simulink model "SIM_EXO_DAL"  (R2021b)
(part 18 of 25)

et753 = t4.*t5.*t7.*1.873025744810486e-7-t4.*t7.*t9.*3.446085442739697e-7;
et754 = t91.*t5684.*t6216.*1.656182742171539e-72;
et755 = t91.*t5824.*t6213.*(-1.656182742171539e-72);
et756 = t5684.*t6230.*(t29-t30).*(-1.656182742171539e-72);
et757 = t5824.*t6222.*(t29-t30).*1.656182742171539e-72;
et758 = t4.*8.79383415291399e-9-t8.*1.262353016789131e-9+(t6401.*(t5808-t6019+t5679.*(t2088-t4743).*3.038581678643136e-64))./2.0;
et759 = t5.*t8.*2.179051830709965e-7-t8.*t72-(t4.*t640)./2.0-t8.*t1496+(t5.*t3443)./2.0-(t9.*t3514)./2.0-(t615.*t6422)./2.0;
et760 = (t6359.*(t5831-t6095+t5679.*(t2088-t4743).*8.081970098144003e-70))./2.0+(t8.*t9.*t1460)./2.0;
et761 = t4.*(-3.403234468928681e-8);
et762 = t202.*1.910352536348279e-6;
et763 = t7.*t8.*5.724235841753608e-8;
et764 = t4.*t190.*1.109465165290797e-6-t9.*t5657.*4.00912737776847e-7+t112.*t5657;
et765 = t5.*t6349.*(-7.01299275e-12)-t9.*t6350.*7.01299275e-12+(t5.*t7042)./2.0+(t9.*t7045)./2.0+t1489.*t5657-(t1426.*t5939)./2.0-(t5658.*t6405)./2.0+(t5662.*t6402)./2.0-(t5939.*t6399)./2.0+(t5940.*t6400)./2.0+(t6422.*t7012)./2.0-(t640.*(t2421-t4158))./2.0-(t5.*t1471.*t5657)./2.0;
et766 = t3.*t8.*t34.*t191.*2.142628988669224e-22;
et767 = t263-t300-t373+t377+t395-t402+t431-t441+t442-t454-t457-t481+t482-t489+t491-t494+t496+t516+t517-t540+t559+t563+t564-t568-t582+t584+t605+t614-t625-t911-t971-t986+t1282-t1670+t4089+t4123+t7221+t7223;
et768 = (t1426.*(-t5881+t5918+t6412+t6414+(t4.*t5824.*t5861.*(t29-t30))./1.316403645856965e+67+(t4.*t91.*t5824.*(t3136-t5691))./1.316403645856965e+67))./2.0;
et769 = t3.*t8.*5.337065020227051e-7-t3.*t5.*t8.*1.873025744810486e-7;
et770 = t5.*t7.*t9.*t18.*(-1.07175327657342e-6);
et771 = t199.*4.620317820983189e-6+t753+t797+t848+t852+t902+t908+t917+t928+t931+t944+t952+t975+t976+t991+t1090+t1122+t1147+t1156+t1194+t1292+t1441+t1816+t2028+t2486+t3416+t3417+t3426+t3429+t3432+t3464+t3465+t3469+t3489+t3498+t3501+t3504+t3510+t3521+t3530+t3535+t3540+t3554+t3571+t3574+t3577+t3578+t3605+t3607+t3637+t3659+t3666+t3694+t3726+t3863+t3960+t4004+t4011+t4015;
et772 = t4134+t4423+t4592+t4780-t5621-t5847-t5849-t5982+t6360-t6362-t6442+t6445-t6451-t6563-t6564+t6879+t7006+t7008+t7022+t7023+t3.*t4.*1.384445455377623e-7;
et773 = t4.*t7.*t34.*t191.*(-5.182094253151392e-22);
et774 = (t6401.*(t5808-t6019+t5679.*(t2088-t4743).*3.038581678643136e-64))./2.0;
et775 = (t6359.*(t5831-t6095+t5679.*(t2088-t4743).*8.081970098144003e-70))./2.0;
et776 = t5888+t5795.*(t2088-t4743).*8.081970098144003e-70;
et777 = t5683.*(t197.*(t29-t30).*9.007199254740992e+15+t3.*(t2444-t2449)).*8.081970098144003e-70;
et778 = t5842+t5795.*(t2088-t4743).*3.038581678643136e-64;
et779 = t5683.*(t197.*(t29-t30).*9.007199254740992e+15+t3.*(t2444-t2449)).*3.038581678643136e-64;
et780 = t201.*8.987911871652987e-9+t202.*6.359001115808088e-7-t1542+t1551+t1627+t1648+t1710+t1732+t1806-t1855+t1922+t1947-t1986+t2002+t2017+t2035-t2062-t2123+t2143-t2181-t2187+t2192-t2196-t2202;
et781 = -t2213-t2289+t2303-t2312+t2314+t2338-t2392+t2397+t2465+t2524-t2530+t2539+t2554+t2556+t2560+t2627+t4279+t4395+t4406+t4416+t4426+t4462-t4469+t4490-t4520+t4545-t4551+t4558-t4559+t4575-t4581+t4588+t4589-t4590-t4591-t4605-t4607-t4614+t4616-t4622+t4626+t4666-t4667-t4669+t4675-t4694+t4695-t4697+t4708-t4724-t4732-t4745+t4747-t4755+t4756+t4782+t4785-t4786;
et782 = t4.*t190.*1.069583140309415e-6-t5.*t201.*1.608000198040319e-13;
et783 = t5.*t202.*(-2.227142959217101e-7)+t9.*t201.*2.10868590222219e-13;
et784 = t19.*t202.*(-1.274380648825446e-6)+t202.*t240+t23.*t1551+t23.*t1627+t5.*t1687-t4.*t5.*t190.*3.746051489620971e-7;
et785 = t4.*t9.*t190.*6.892170885479394e-7-t8.*t9.*t190.*3.546806877605634e-13;
et786 = t4.*t19.*t190.*(-2.143506553146841e-6)+t5.*t9.*t202.*8.376559107229145e-7;
et787 = t4.*t34.*t191.*(-3.795202701448175e-22);
et788 = t8.*t34.*t191.*2.95048074153502e-22;
et789 = t19.*t23.*t196.*(-4.188279553614573e-7)+t4.*t5.*t9.*t190.*1.408936125616489e-6;
et790 = t5.*t8.*t17.*t190.*(-2.7046541903611e-13);
et791 = t3.*t4.*t34.*t191.*5.099405807101157e-25;
et792 = t5.*t9.*t23.*t196.*(-6.371903244127231e-7);
et793 = t3.*t8.*t34.*t191.*3.607859943485489e-23;
et794 = t4.*t7.*t34.*t191.*4.962704675595027e-22;
et795 = t5.*t8.*t34.*t191.*3.738830062544659e-22;
et796 = t7.*t8.*t34.*t191.*6.383525886533628e-22;
et797 = t8.*t9.*t34.*t191.*2.032139097819379e-22;
et798 = t3.*t4.*t5.*t34.*t191.*(-9.123193089563036e-30);
et799 = t3.*t4.*t9.*t34.*t191.*1.196389694146674e-29;
et800 = t3.*t5.*t8.*t34.*t191.*(-1.263597807995354e-23);
et801 = t4.*t5.*t7.*t34.*t191.*6.288707183017346e-22;
et802 = t3.*t8.*t9.*t34.*t191.*2.324829770052718e-23;
et803 = t4.*t7.*t9.*t34.*t191.*3.418055254602648e-22;
et804 = t3.*t8.*t19.*t34.*t191.*(-7.230360259287513e-23);
et805 = t3.*t4.*t5.*t7.*t34.*t191.*(-2.125369829239315e-23);
et806 = t3.*t5.*t8.*t9.*t34.*t191.*4.752547061531711e-23;
et807 = t5961-t6215-t6473+(t91.*t5824.*(t5670+t4.*(t1458-t5665)))./1.316403645856965e+67+(t5824.*t6103.*(t29-t30))./1.316403645856965e+67;
et808 = (t5822.*t6230.*(t29-t30))./1.316403645856965e+67;
et809 = t5889+t5795.*(t2088-t4743).*5.344156668414146e-72;
et810 = t5683.*(t197.*(t29-t30).*9.007199254740992e+15+t3.*(t2444-t2449)).*5.344156668414146e-72;
et811 = t5888+t5795.*(t2088-t4743).*8.081970098144003e-70;
et812 = t5683.*(t197.*(t29-t30).*9.007199254740992e+15+t3.*(t2444-t2449)).*8.081970098144003e-70;
et813 = t5892+t5795.*(t2088-t4743).*7.671525497590686e-73;
et814 = t5683.*(t197.*(t29-t30).*9.007199254740992e+15+t3.*(t2444-t2449)).*7.671525497590686e-73;
et815 = t6008+t6123-t6672+(t5684.*t6468.*(t29-t30))./1.316403645856965e+67-(t5.*t91.*t5824.*t6216)./1.316403645856965e+67;
et816 = (t5.*t5824.*t6230.*(t29-t30))./1.316403645856965e+67;
et817 = t5882+t5795.*(t2088-t4743).*1.879526485671887e-68;
et818 = t5683.*(t197.*(t29-t30).*9.007199254740992e+15+t3.*(t2444-t2449)).*1.879526485671887e-68;
et819 = t5883+t5795.*(t2088-t4743).*4.121912899099809e-68;
et820 = t5683.*(t197.*(t29-t30).*9.007199254740992e+15+t3.*(t2444-t2449)).*4.121912899099809e-68;
et821 = t741+t868+t1568+t1834-t3274-t3391-t3440+t3874+t3891+t4348+t5259+t5742+t5757-t5.*t8.*1.133811468776912e-7;
et822 = t5.*t201.*(-6.364473664374288e-6)+t8.*t3365+t8.*t3449;
et823 = t4.*t5.*t7.*(-1.907069379620846e-7);
et824 = t8.*t9.*t190.*(-6.800564119502148e-6);
et825 = t3.*t4.*t5.*t34.*t191.*(-7.138318981153782e-22);
et826 = t199.*(-2.737706926505492e-6)+t1541+t1570+t1607-t1609-t1616+t1656+t1747-t1783+t1792-t1805+t1908-t2795+t4181+t4221-t4228+t4342-t4344+t4345-t4403+t4413-t4431-t4495+t4501-t4502+t4509+t4919+t4983-t5769+t5921+t5922+t6119+t6406-t6407+t6443-t6477+t6489+t6593-t6594-t7051-t7054;
et827 = -t7088+t7091+t7114-t7115+t7174+t7261-t7322+(t5658.*(et809+et810))./2.0+(t6776.*(t6313+(t91.*t5824.*(t6218+t5.*(t3136-t5691)))./1.316403645856965e+67+(t5824.*t6470.*(t29-t30))./1.316403645856965e+67))./2.0;
et828 = (t4119.*(et811+et812))./2.0+(t5662.*(et813+et814))./2.0+(t7027.*(et815+et816))./2.0+(t5940.*(et817+et818))./2.0+(t5939.*(et819+et820))./2.0+(t318.*(et821+et822+et823+et824+et825))./2.0-t4.*t17.*t190.*2.170136264005124e-9;
et829 = t8.*t34.*t191.*(-3.477878712271355e-22);
et830 = t4.*t7.*t34.*t191.*9.787964718254394e-24;
et831 = dq5.*((t6359.*(et776+et777))./2.0+(t6401.*(et778+et779))./2.0)-dq1.*(et780+et781+et782+et783+et784+et785+et786+et787+et788+et789+et790+et791+et792+et793+et794+et795+et796+et797+et798+et799+et800+et801+et802+et803+et804+et805+et806)+dq6.*(t3142-t4099-t4103+t4810-t4904+t7066+t7074+t7307+t7308+t7376+t7377+t7380+t7427+t7428+t7447+t7448+t7468+t7477+t7491+t7492+t7493);
et832 = -dq3.*(t922+t934+t940+t989+t1039+t1050+t1056+t1069+t1083+t1099+t1106+t1133+t1150+t1177+t1179+t1185+t1191+t1196+t1205+t1221+t1225+t1233+t1250+t1253+t1273+t1274+t1306+t1316+t1322+t1330+t1331+t1337+t1342+t1348+t1353+t1379+t1391+t1402+t1407+t1411+t1413+t1419+t1423+t1436+t1443+t1445+t1454+t1457+t1486+t1487+t1767+t1827+t1873+t1992+t2130+t2180+t2474+t2481+t5.*t7274.*1.40259855e-11-t9.*t7276.*1.40259855e-11+t1426.*(et807+et808))+dq2.*(et826+et827+et828+et829+et830);
et833 = -dq4.*(t290+t357+t406+t411+t418+t423+t424+t429+t440+t449+t479+t480+t483+t488+t492+t532+t540+t545+t580+t581+t590+t604+t611+t618+t623+t911+t971+t986+t1324+t1670+t4100+t4132+t7143+t7222+t7224);
et834 = -t235+t315+t413+t539+t543+t567+t6081-t6167+t6182+t6521+t6537-t6677+t5704.*t5784+t91.*t5684.*(t6218+t5.*(t3136-t5691)).*1.015171749786156e-71;
et835 = t5684.*t6468.*(t29-t30).*5.517689141340903e-72;
et836 = t5684.*t6470.*(t29-t30).*1.015171749786156e-71;
et837 = t5.*t91.*t5824.*t6216.*(-5.517689141340903e-72);
et838 = t5.*t5824.*t6230.*(t29-t30).*5.517689141340903e-72;
et839 = t284-t311+t391-t463+t534+t5947-t6009.*1.40259855e-11+t6013.*7.26350610236655e-5-t6194+t6449+t6454-t6513+t6544+t6551;
et840 = t91.*t5684.*(t6218+t5.*(t3136-t5691)).*1.065477564130357e-78-t4.*t7.*t9.*1.07175327657342e-6;
et841 = t5824.*t6222.*(t29-t30).*5.517689141340903e-72;
et842 = t5684.*t6470.*(t29-t30).*1.065477564130357e-78;
et843 = t741+t868+t1568+t1834-t3274-t3391-t3440+t3874+t3891+t4348+t5259+t5742+t5757-t5.*t8.*1.133811468776912e-7;
et844 = t5.*t201.*(-6.364473664374288e-6)+t8.*t3365+t8.*t3449;
et845 = t4.*t5.*t7.*(-1.907069379620846e-7);
et846 = t8.*t9.*t190.*(-6.800564119502148e-6);
et847 = t3.*t4.*t5.*t34.*t191.*(-7.138318981153782e-22);
et848 = dq3.*(t3142+t4108+t4115+t4810+t4984+t7066+t7074+t7307+t7308+t7414+t7442+t7444+t7504+(t6821.*(et834+et835+et836+et837+et838))./2.0+(t7130.*(et839+et840+et841+et842))./2.0)-dq4.*(t622+t632+t712+t1503+t1523+t6941+t7059+t7081+t7136+t7137+t7201+t7203+t7272+t7273)+dq5.*(-t72+t112+t616+t619-t1489+t1496)+dq6.*(-t7459-t7501+t7502+t7508-t7541-t7542+t638.*t6821+t594.*t7129+t600.*t7130-t1460.*t7130+t1471.*t7129)+dq2.*(t5797+t5926+t5928+t5937+t5938+t6271+t7231+t7235-t7271-t7343+t7344+(t6821.*(et843+et844+et845+et846+et847))./2.0);
et849 = -dq1.*(t684+t781+t792+t803+t826+t832+t875+t893+t912+t915+t1088+t1201+t1612+t1734+t1740+t1814+t1833+t1968+t1997+t2004+t2069+t2115+t2133+t2267+t3338+t3375+t3390+t3392+t3400+t3420+t3422+t3435+t3437+t3439+t3446+t3458+t3474+t3483+t3491+t3547+t3556+t3610+t3662+t3706+t3755+t3763+t3792+t3822+t3831+t3852+t3873+t3951+t3957+t3979+t3993+t4249+t4304+t4347+t4447+t4527+t4587+t7257-t7341-t7342+t7405-t7431-t7434);
et850 = t5889+t5795.*(t2088-t4743).*5.344156668414146e-72;
et851 = t5683.*(t197.*(t29-t30).*9.007199254740992e+15+t3.*(t2444-t2449)).*5.344156668414146e-72;
et852 = t5888+t5795.*(t2088-t4743).*8.081970098144003e-70;
et853 = t5683.*(t197.*(t29-t30).*9.007199254740992e+15+t3.*(t2444-t2449)).*8.081970098144003e-70;
et854 = t5892+t5795.*(t2088-t4743).*7.671525497590686e-73;
et855 = t5683.*(t197.*(t29-t30).*9.007199254740992e+15+t3.*(t2444-t2449)).*7.671525497590686e-73;
et856 = -t231+t275+t469+t553+t6074+t6175-t6676+t5.*t6536+t5684.*t6468.*(t29-t30).*5.520609140571798e-70;
et857 = t5.*t91.*t5824.*t6216.*(-5.520609140571798e-70);
et858 = t5882+t5795.*(t2088-t4743).*1.879526485671887e-68;
et859 = t5683.*(t197.*(t29-t30).*9.007199254740992e+15+t3.*(t2444-t2449)).*1.879526485671887e-68;
et860 = t5883+t5795.*(t2088-t4743).*4.121912899099809e-68;
et861 = t5683.*(t197.*(t29-t30).*9.007199254740992e+15+t3.*(t2444-t2449)).*4.121912899099809e-68;
et862 = -dq1.*(t7558-t7574+dq6.*t7104+dq4.*t7256-dq3.*t7595)+dq5.*(-dq6.*(et735+et736+et737)+dq3.*(et748+et749+et750+et751+et752+et753+et754+et755+et756+et757)+dq4.*(et758+et759+et760)+dq2.*(et761+et762+et763+et764+et765+et766));
et863 = -dq4.*(t5825+t7258+dq2.*(et771+et772+et773)+dq6.*(t622-t624-t681+t1503+t1523+t7059+t7206+t7272+t7273+t7348-t7350+t7367-t7369+t7371-t7485+t7487-t7490+t4.*t9.*(t5709-t6255+t6282+t6296-t7003+t6216.*(t6218+t5.*(t3136-t5691)).*1.40259855e-11).*(3.0./1.0e+3))-dq3.*(et767+et768+et769+et770)-dq5.*(et774+et775))+dq3.*(et831+et832+et833)+dq6.*(et848+et849);
et864 = dq2.*(-t7557-t7558+dq4.*t7572+dq6.*t7597+dq3.*(-t5769+t5921+t5922+t5958-t5960+t5974+t5978+t6119+t6202+t6203+t6209+t6210-t6329+t6330+t6406-t6407+t6443-t6477+t6489+t6593-t6594-t7102+t7156-t7158+t7217+t7277+t7279+t7300+t7321+t7435+t7437+t7455+(t5658.*(et850+et851))./2.0+(t4119.*(et852+et853))./2.0+(t5662.*(et854+et855))./2.0+(t6462.*(et856+et857))./2.0+(t5940.*(et858+et859))./2.0+(t5939.*(et860+et861))./2.0));
et865 = t6191.*(-2.179051830709965e-7)+t6197.*4.00912737776847e-7+t6930.*4.00912737776847e-7+t6937.*4.00912737776847e-7;
et866 = t6939.*(-2.179051830709965e-7)-t7459-t7501+t7502+t7508-t7541-t7542+t6216.*(t6218+t5.*(t3136-t5691)).*2.179051830709965e-7+(t9.*(-t6235+t6248+t6952+t6983-t6989+t6216.*(t6218+t5.*(t3136-t5691)).*1.744166498897461e-6))./2.0-(t5.*t7366)./2.0+(t638.*t6821)./2.0;
et867 = (t594.*t7129)./2.0+(t600.*t7130)./2.0-(t1460.*t7130)./2.0+(t1471.*t7129)./2.0+(t9.*(-t5744+t6232+t6248+t6303+t6322+t6952+t6960+t6983+t6991))./2.0+(t5.*(t6197.*3.383302988283333e-6-t6231+t6954+t6985-t6990+t6216.*(t6218+t5.*(t3136-t5691)).*1.246862701090643e-6))./2.0;
et868 = ((t4148+t5.*(t2421-t4158)).*(-t6235+t6248+t6952+t6983-t6989+t6216.*(t6218+t5.*(t3136-t5691)).*1.744166498897461e-6))./2.0-(t5657.*t7331)./2.0-(t5872.*t7366)./2.0-(t6462.*t7133)./2.0+(t6463.*t7134)./2.0+(t6462.*t7204)./2.0-(t6821.*t7098)./2.0+(t7032.*t7129)./2.0-(t7033.*t7130)./2.0-(t7082.*t7130)./2.0+(t7085.*t7129)./2.0+((t4148+t5.*(t2421-t4158)).*(-t5744+t6232+t6248+t6303+t6322+t6952+t6960+t6983+t6991))./2.0;
et869 = (t6136.*(t6197.*1.33637579258949e-4-t6225+t6944+t6975-t6986+t6216.*(t6218+t5.*(t3136-t5691)).*7.26350610236655e-5))./2.0+(t6463.*(t5709-t6255+t6282+t6296-t7003+t6216.*(t6218+t5.*(t3136-t5691)).*1.40259855e-11))./2.0;
et870 = (t5872.*(t6197.*3.383302988283333e-6-t6231+t6954+t6985-t6990+t6216.*(t6218+t5.*(t3136-t5691)).*1.246862701090643e-6))./2.0;
et871 = (t7130.*(-t6235+t6248+t6952+t6983-t6989+t6216.*(t6218+t5.*(t3136-t5691)).*1.744166498897461e-6))./2.0-(t6821.*t7331)./2.0-(t7129.*t7366)./2.0+(t7130.*(-t5744+t6232+t6248+t6303+t6322+t6952+t6960+t6983+t6991))./2.0;
et872 = (t7129.*(t6197.*3.383302988283333e-6-t6231+t6954+t6985-t6990+t6216.*(t6218+t5.*(t3136-t5691)).*1.246862701090643e-6))./2.0;
et873 = t6313+(t91.*t5824.*(t6218+t5.*(t3136-t5691)))./1.316403645856965e+67+(t5824.*t6470.*(t29-t30))./1.316403645856965e+67;
et874 = (t5709-t6255+t6282+t6296-t7003+t6216.*(t6218+t5.*(t3136-t5691)).*1.40259855e-11)./2.0;
et875 = t7453+t7529+t7530+t7552+t7562+t7563+(t7133.*(-t6729+t5784.*(t4148+t5.*(t2421-t4158))+(t5824.*t6468.*(t29-t30))./1.316403645856965e+67))./2.0;
et876 = t7204.*(-t6729+t5784.*(t4148+t5.*(t2421-t4158))+(t5824.*t6468.*(t29-t30))./1.316403645856965e+67).*(-1.0./2.0);
et877 = (t7134.*(t6313+(t91.*t5824.*(t6218+t5.*(t3136-t5691)))./1.316403645856965e+67+(t5824.*t6470.*(t29-t30))./1.316403645856965e+67))./2.0;
et878 = (t1427.*(-t6235+t6248+t6952+t6983-t6989+t6216.*(t6218+t5.*(t3136-t5691)).*1.744166498897461e-6))./2.0+(t318.*t7331)./2.0-(t1429.*t7366)./2.0+(t6821.*t7309)./2.0-(t7124.*t7130)./2.0-(t7130.*t7267)./2.0-(t7129.*t7269)./2.0;
et879 = (t7129.*(t305-t319+t322+t336+t6345+t6807+t6818-t5.*t7.*t8.*2.908151843953269e-6-t7.*t8.*t9.*1.07175327657342e-6))./2.0+(t1427.*(-t5744+t6232+t6248+t6303+t6322+t6952+t6960+t6983+t6991))./2.0+et873.*et874;
et880 = ((t6005-t6486+(t5824.*t6230.*(t29-t30))./1.316403645856965e+67).*(t6197.*1.33637579258949e-4-t6225+t6944+t6975-t6986+t6216.*(t6218+t5.*(t3136-t5691)).*7.26350610236655e-5))./2.0;
et881 = (t1429.*(t6197.*3.383302988283333e-6-t6231+t6954+t6985-t6990+t6216.*(t6218+t5.*(t3136-t5691)).*1.246862701090643e-6))./2.0;
et882 = t738+t910+t930+t1019+t1077+t1212+t1659+t1835+t1938+t2052+t3457+t3479+t3542+t3584+t3612+t3667+t3732+t3875+t3922+t3968+t4286+t4349+t4370+t4553-t4.*t5.*1.043021220661002e-7;
et883 = t4.*t9.*(-5.669057343884558e-8)+t8.*t1798+t8.*t2083+t8.*t4183+t8.*t4208+t8.*t4259+t8.*t4337-(t6821.*t7297)./2.0+(t7129.*t7141)./2.0-(t7130.*t7140)./2.0+(t7130.*t7244)./2.0+(t7129.*t7248)./2.0;
et884 = t2.*t3.*t5.*(-3.337218585173762e-6);
et885 = t2.*t4.*t5.*(-3.65040710056658e-6);
et886 = t2.*t3.*t9.*6.139979878798348e-6;
et887 = t3.*t5.*t6.*8.090164539562037e-7;
et888 = t2.*t4.*t9.*(-1.984079208716435e-6);
et889 = t4.*t5.*t6.*8.849403575532204e-7;
et890 = t3.*t6.*t9.*(-1.488468502176114e-6);
et891 = t4.*t6.*t9.*4.809851931591181e-7;
et892 = t4.*t5.*t190.*3.400282059751074e-6;
et893 = t2.*t5.*t196.*(-4.809851931591181e-7);
et894 = t4.*t9.*t190.*1.848130565348858e-6;
et895 = t2.*t9.*t196.*8.849403575532204e-7;
et896 = t5.*t6.*t196.*(-1.984079208716435e-6);
et897 = t2.*t5.*t202.*8.849403575532204e-7;
et898 = t6.*t9.*t196.*3.65040710056658e-6;
et899 = t2.*t9.*t202.*4.809851931591181e-7;
et900 = t5.*t6.*t202.*3.65040710056658e-6;
et901 = t6.*t9.*t202.*1.984079208716435e-6;
et902 = t5.*t6.*t7.*t8.*(-1.488468502176114e-6);
C_dq = ft_17({dq1,dq2,dq3,dq4,dq5,dq6,et294,et295,et296,et341,et342,et343,et627,et628,et629,et630,et732,et733,et734,et862,et863,et864,et865,et866,et867,et868,et869,et870,et871,et872,et875,et876,et877,et878,et879,et880,et881,et882,et883,et884,et885,et886,et887,et888,et889,et890,et891,et892,et893,et894,et895,et896,et897,et898,et899,et900,et901,et902,t1004,t1016,t1031,t1061,t1075,t1081,t1095,t1101,t1108,t113,t1144,t115,t1152,t1155,t1170,t1171,t1174,t1184,t1193,t1203,t1207,t1213,t1215,t1224,t1227,t1245,t125,t1254,t1258,t1285,t1288,t1300,t1301,t131,t132,t1323,t1333,t1344,t1345,t1365,t1377,t1380,t1383,t1388,t1409,t1427,t1428,t1429,t144,t1440,t1458,t148,t1489,t150,t1503,t1508,t1523,t1537,t1540,t156,t158,t1593,t1621,t1622,t1642,t1661,t1672,t1692,t17,t1704,t171,t1715,t1719,t1721,t1731,t1759,t1769,t1770,t1775,t1777,t18,t1831,t1847,t185,t1858,t1870,t19,t190,t191,t196,t1977,t1981,t1984,t199,t2,t2014,t2034,t2043,t2096,t2121,t2132,t2150,t2165,t2177,t2184,t2203,t2236,t2333,t2341,t2383,t2390,t2395,t24,t2421,t2546,t257,t258,t277,t278,t287,t29,t3,t30,t302,t309,t3136,t3142,t318,t3321,t34,t3407,t3409,t3430,t3444,t3450,t3463,t3468,t3475,t3485,t3490,t3496,t3499,t3507,t3513,t3515,t3522,t3523,t3526,t3531,t3543,t356,t3569,t358,t3583,t3585,t3606,t361,t3618,t3658,t371,t3719,t372,t3734,t3738,t374,t3757,t3788,t379,t3843,t3869,t3871,t3992,t4,t4099,t4103,t4148,t4153,t4158,t4179,t4185,t4190,t422,t4230,t4232,t4254,t4255,t427,t428,t4317,t433,t434,t436,t4369,t4396,t4397,t4412,t4417,t4419,t4420,t4428,t4429,t4436,t444,t4440,t445,t4478,t448,t4485,t4506,t4519,t452,t4522,t453,t4530,t4541,t4549,t4556,t4557,t4568,t4572,t458,t4596,t460,t4619,t4625,t4648,t4656,t4660,t4727,t4733,t4739,t475,t477,t4810,t485,t486,t4904,t493,t5,t508,t510,t512,t514,t520,t522,t524,t5275,t533,t535,t547,t561,t5665,t5666,t5670,t5676,t5691,t5709,t5718,t5730,t5738,t5744,t5784,t5822,t5824,t5845,t586,t5861,t587,t5878,t5905,t592,t5942,t5943,t5944,t5951,t5954,t596,t5961,t5967,t5973,t6,t6005,t6026,t603,t6035,t6037,t6042,t6044,t6046,t6047,t6048,t6053,t6056,t6060,t610,t6103,t6118,t612,t6142,t6145,t6146,t6147,t6152,t6155,t6158,t6162,t6164,t6165,t6170,t6171,t6177,t6179,t6183,t6189,t6195,t6196,t6197,t620,t621,t6213,t6215,t6216,t6218,t622,t6220,t6226,t6230,t6231,t6232,t6235,t6239,t6244,t6248,t6249,t6252,t6255,t6276,t6282,t6289,t6293,t6296,t6303,t6307,t6312,t6313,t632,t6322,t6352,t6465,t6468,t6470,t6473,t6486,t6487,t6546,t6548,t6557,t6562,t6604,t6605,t6607,t6648,t6656,t6711,t6714,t6715,t6721,t6724,t6727,t6729,t6738,t6743,t6746,t6747,t6753,t6756,t6758,t6821,t6831,t6838,t6841,t6842,t6844,t6847,t6849,t6851,t6856,t6859,t6860,t6865,t6884,t6888,t6890,t6891,t6892,t6894,t6898,t6903,t6909,t6911,t6914,t6915,t6916,t6918,t6921,t6922,t6924,t6928,t6935,t6936,t6946,t6952,t6953,t6954,t6960,t6977,t6983,t6984,t6985,t6989,t6990,t6991,t6994,t7,t7000,t7003,t7026,t7035,t7036,t7039,t7040,t7084,t7086,t7087,t7095,t7096,t7100,t7103,t7104,t712,t7127,t7128,t7129,t7130,t7133,t7134,t7194,t72,t7204,t7206,t7207,t7208,t724,t7242,t7243,t7245,t7246,t7247,t7254,t7255,t7268,t7270,t7274,t7276,t73,t7327,t7331,t7332,t7336,t7340,t7346,t7348,t7349,t7350,t7362,t7363,t7366,t7367,t7368,t7369,t7371,t7372,t7373,t7374,t7375,t7376,t7377,t7378,t7379,t7380,t7381,t7382,t7383,t7384,t7385,t7390,t7391,t7392,t7393,t7394,t7395,t7396,t7398,t7399,t7402,t7403,t742,t7423,t7425,t7426,t7427,t7428,t7429,t7430,t7433,t7439,t7440,t7446,t7447,t7448,t7453,t7459,t7463,t7468,t7476,t7477,t7481,t7482,t7485,t7486,t7487,t7488,t7490,t7491,t7492,t7493,t7496,t7498,t7499,t7500,t7501,t7503,t7507,t7509,t7510,t7511,t7512,t7513,t7515,t7516,t7517,t7519,t7521,t7522,t7523,t7524,t7525,t7526,t7527,t7529,t7530,t7531,t7533,t7534,t7536,t7537,t7538,t7541,t7542,t7543,t7546,t7548,t7549,t7550,t7552,t7554,t7555,t7562,t7563,t7565,t7587,t7597,t7599,t8,t825,t827,t845,t866,t869,t874,t877,t881,t899,t9,t90,t903,t91,t919,t926,t932,t947,t957,t958,t968,t970,t972,t984,t985,t998});
end
function C_dq = ft_17(ct)
dq1 = ct{1};
dq2 = ct{2};
dq3 = ct{3};
dq4 = ct{4};
dq5 = ct{5};
dq6 = ct{6};
et294 = ct{7};
et295 = ct{8};
et296 = ct{9};
et341 = ct{10};
et342 = ct{11};
et343 = ct{12};
et627 = ct{13};
et628 = ct{14};
et629 = ct{15};
et630 = ct{16};
et732 = ct{17};
et733 = ct{18};
et734 = ct{19};
et862 = ct{20};
et863 = ct{21};
et864 = ct{22};
et865 = ct{23};
et866 = ct{24};
et867 = ct{25};
et868 = ct{26};
et869 = ct{27};
et870 = ct{28};
et871 = ct{29};
et872 = ct{30};
et875 = ct{31};
et876 = ct{32};
et877 = ct{33};
et878 = ct{34};
et879 = ct{35};
et880 = ct{36};
et881 = ct{37};
et882 = ct{38};
et883 = ct{39};
et884 = ct{40};
et885 = ct{41};
et886 = ct{42};
et887 = ct{43};
et888 = ct{44};
et889 = ct{45};
et890 = ct{46};
et891 = ct{47};
et892 = ct{48};
et893 = ct{49};
et894 = ct{50};
et895 = ct{51};
et896 = ct{52};
et897 = ct{53};
et898 = ct{54};
et899 = ct{55};
et900 = ct{56};
et901 = ct{57};
et902 = ct{58};
t1004 = ct{59};
t1016 = ct{60};
t1031 = ct{61};
t1061 = ct{62};
t1075 = ct{63};
t1081 = ct{64};
t1095 = ct{65};
t1101 = ct{66};
t1108 = ct{67};
t113 = ct{68};
t1144 = ct{69};
t115 = ct{70};
t1152 = ct{71};
t1155 = ct{72};
t1170 = ct{73};
t1171 = ct{74};
t1174 = ct{75};
t1184 = ct{76};
t1193 = ct{77};
t1203 = ct{78};
t1207 = ct{79};
t1213 = ct{80};
t1215 = ct{81};
t1224 = ct{82};
t1227 = ct{83};
t1245 = ct{84};
t125 = ct{85};
t1254 = ct{86};
t1258 = ct{87};
t1285 = ct{88};
t1288 = ct{89};
t1300 = ct{90};
t1301 = ct{91};
t131 = ct{92};
t132 = ct{93};
t1323 = ct{94};
t1333 = ct{95};
t1344 = ct{96};
t1345 = ct{97};
t1365 = ct{98};
t1377 = ct{99};
t1380 = ct{100};
t1383 = ct{101};
t1388 = ct{102};
t1409 = ct{103};
t1427 = ct{104};
t1428 = ct{105};
t1429 = ct{106};
t144 = ct{107};
t1440 = ct{108};
t1458 = ct{109};
t148 = ct{110};
t1489 = ct{111};
t150 = ct{112};
t1503 = ct{113};
t1508 = ct{114};
t1523 = ct{115};
t1537 = ct{116};
t1540 = ct{117};
t156 = ct{118};
t158 = ct{119};
t1593 = ct{120};
t1621 = ct{121};
t1622 = ct{122};
t1642 = ct{123};
t1661 = ct{124};
t1672 = ct{125};
t1692 = ct{126};
t17 = ct{127};
t1704 = ct{128};
t171 = ct{129};
t1715 = ct{130};
t1719 = ct{131};
t1721 = ct{132};
t1731 = ct{133};
t1759 = ct{134};
t1769 = ct{135};
t1770 = ct{136};
t1775 = ct{137};
t1777 = ct{138};
t18 = ct{139};
t1831 = ct{140};
t1847 = ct{141};
t185 = ct{142};
t1858 = ct{143};
t1870 = ct{144};
t19 = ct{145};
t190 = ct{146};
t191 = ct{147};
t196 = ct{148};
t1977 = ct{149};
t1981 = ct{150};
t1984 = ct{151};
t199 = ct{152};
t2 = ct{153};
t2014 = ct{154};
t2034 = ct{155};
t2043 = ct{156};
t2096 = ct{157};
t2121 = ct{158};
t2132 = ct{159};
t2150 = ct{160};
t2165 = ct{161};
t2177 = ct{162};
t2184 = ct{163};
t2203 = ct{164};
t2236 = ct{165};
t2333 = ct{166};
t2341 = ct{167};
t2383 = ct{168};
t2390 = ct{169};
t2395 = ct{170};
t24 = ct{171};
t2421 = ct{172};
t2546 = ct{173};
t257 = ct{174};
t258 = ct{175};
t277 = ct{176};
t278 = ct{177};
t287 = ct{178};
t29 = ct{179};
t3 = ct{180};
t30 = ct{181};
t302 = ct{182};
t309 = ct{183};
t3136 = ct{184};
t3142 = ct{185};
t318 = ct{186};
t3321 = ct{187};
t34 = ct{188};
t3407 = ct{189};
t3409 = ct{190};
t3430 = ct{191};
t3444 = ct{192};
t3450 = ct{193};
t3463 = ct{194};
t3468 = ct{195};
t3475 = ct{196};
t3485 = ct{197};
t3490 = ct{198};
t3496 = ct{199};
t3499 = ct{200};
t3507 = ct{201};
t3513 = ct{202};
t3515 = ct{203};
t3522 = ct{204};
t3523 = ct{205};
t3526 = ct{206};
t3531 = ct{207};
t3543 = ct{208};
t356 = ct{209};
t3569 = ct{210};
t358 = ct{211};
t3583 = ct{212};
t3585 = ct{213};
t3606 = ct{214};
t361 = ct{215};
t3618 = ct{216};
t3658 = ct{217};
t371 = ct{218};
t3719 = ct{219};
t372 = ct{220};
t3734 = ct{221};
t3738 = ct{222};
t374 = ct{223};
t3757 = ct{224};
t3788 = ct{225};
t379 = ct{226};
t3843 = ct{227};
t3869 = ct{228};
t3871 = ct{229};
t3992 = ct{230};
t4 = ct{231};
t4099 = ct{232};
t4103 = ct{233};
t4148 = ct{234};
t4153 = ct{235};
t4158 = ct{236};
t4179 = ct{237};
t4185 = ct{238};
t4190 = ct{239};
t422 = ct{240};
t4230 = ct{241};
t4232 = ct{242};
t4254 = ct{243};
t4255 = ct{244};
t427 = ct{245};
t428 = ct{246};
t4317 = ct{247};
t433 = ct{248};
t434 = ct{249};
t436 = ct{250};
t4369 = ct{251};
t4396 = ct{252};
t4397 = ct{253};
t4412 = ct{254};
t4417 = ct{255};
t4419 = ct{256};
t4420 = ct{257};
t4428 = ct{258};
t4429 = ct{259};
t4436 = ct{260};
t444 = ct{261};
t4440 = ct{262};
t445 = ct{263};
t4478 = ct{264};
t448 = ct{265};
t4485 = ct{266};
t4506 = ct{267};
t4519 = ct{268};
t452 = ct{269};
t4522 = ct{270};
t453 = ct{271};
t4530 = ct{272};
t4541 = ct{273};
t4549 = ct{274};
t4556 = ct{275};
t4557 = ct{276};
t4568 = ct{277};
t4572 = ct{278};
t458 = ct{279};
t4596 = ct{280};
t460 = ct{281};
t4619 = ct{282};
t4625 = ct{283};
t4648 = ct{284};
t4656 = ct{285};
t4660 = ct{286};
t4727 = ct{287};
t4733 = ct{288};
t4739 = ct{289};
t475 = ct{290};
t477 = ct{291};
t4810 = ct{292};
t485 = ct{293};
t486 = ct{294};
t4904 = ct{295};
t493 = ct{296};
t5 = ct{297};
t508 = ct{298};
t510 = ct{299};
t512 = ct{300};
t514 = ct{301};
t520 = ct{302};
t522 = ct{303};
t524 = ct{304};
t5275 = ct{305};
t533 = ct{306};
t535 = ct{307};
t547 = ct{308};
t561 = ct{309};
t5665 = ct{310};
t5666 = ct{311};
t5670 = ct{312};
t5676 = ct{313};
t5691 = ct{314};
t5709 = ct{315};
t5718 = ct{316};
t5730 = ct{317};
t5738 = ct{318};
t5744 = ct{319};
t5784 = ct{320};
t5822 = ct{321};
t5824 = ct{322};
t5845 = ct{323};
t586 = ct{324};
t5861 = ct{325};
t587 = ct{326};
t5878 = ct{327};
t5905 = ct{328};
t592 = ct{329};
t5942 = ct{330};
t5943 = ct{331};
t5944 = ct{332};
t5951 = ct{333};
t5954 = ct{334};
t596 = ct{335};
t5961 = ct{336};
t5967 = ct{337};
t5973 = ct{338};
t6 = ct{339};
t6005 = ct{340};
t6026 = ct{341};
t603 = ct{342};
t6035 = ct{343};
t6037 = ct{344};
t6042 = ct{345};
t6044 = ct{346};
t6046 = ct{347};
t6047 = ct{348};
t6048 = ct{349};
t6053 = ct{350};
t6056 = ct{351};
t6060 = ct{352};
t610 = ct{353};
t6103 = ct{354};
t6118 = ct{355};
t612 = ct{356};
t6142 = ct{357};
t6145 = ct{358};
t6146 = ct{359};
t6147 = ct{360};
t6152 = ct{361};
t6155 = ct{362};
t6158 = ct{363};
t6162 = ct{364};
t6164 = ct{365};
t6165 = ct{366};
t6170 = ct{367};
t6171 = ct{368};
t6177 = ct{369};
t6179 = ct{370};
t6183 = ct{371};
t6189 = ct{372};
t6195 = ct{373};
t6196 = ct{374};
t6197 = ct{375};
t620 = ct{376};
t621 = ct{377};
t6213 = ct{378};
t6215 = ct{379};
t6216 = ct{380};
t6218 = ct{381};
t622 = ct{382};
t6220 = ct{383};
t6226 = ct{384};
t6230 = ct{385};
t6231 = ct{386};
t6232 = ct{387};
t6235 = ct{388};
t6239 = ct{389};
t6244 = ct{390};
t6248 = ct{391};
t6249 = ct{392};
t6252 = ct{393};
t6255 = ct{394};
t6276 = ct{395};
t6282 = ct{396};
t6289 = ct{397};
t6293 = ct{398};
t6296 = ct{399};
t6303 = ct{400};
t6307 = ct{401};
t6312 = ct{402};
t6313 = ct{403};
t632 = ct{404};
t6322 = ct{405};
t6352 = ct{406};
t6465 = ct{407};
t6468 = ct{408};
t6470 = ct{409};
t6473 = ct{410};
t6486 = ct{411};
t6487 = ct{412};
t6546 = ct{413};
t6548 = ct{414};
t6557 = ct{415};
t6562 = ct{416};
t6604 = ct{417};
t6605 = ct{418};
t6607 = ct{419};
t6648 = ct{420};
t6656 = ct{421};
t6711 = ct{422};
t6714 = ct{423};
t6715 = ct{424};
t6721 = ct{425};
t6724 = ct{426};
t6727 = ct{427};
t6729 = ct{428};
t6738 = ct{429};
t6743 = ct{430};
t6746 = ct{431};
t6747 = ct{432};
t6753 = ct{433};
t6756 = ct{434};
t6758 = ct{435};
t6821 = ct{436};
t6831 = ct{437};
t6838 = ct{438};
t6841 = ct{439};
t6842 = ct{440};
t6844 = ct{441};
t6847 = ct{442};
t6849 = ct{443};
t6851 = ct{444};
t6856 = ct{445};
t6859 = ct{446};
t6860 = ct{447};
t6865 = ct{448};
t6884 = ct{449};
t6888 = ct{450};
t6890 = ct{451};
t6891 = ct{452};
t6892 = ct{453};
t6894 = ct{454};
t6898 = ct{455};
t6903 = ct{456};
t6909 = ct{457};
t6911 = ct{458};
t6914 = ct{459};
t6915 = ct{460};
t6916 = ct{461};
t6918 = ct{462};
t6921 = ct{463};
t6922 = ct{464};
t6924 = ct{465};
t6928 = ct{466};
t6935 = ct{467};
t6936 = ct{468};
t6946 = ct{469};
t6952 = ct{470};
t6953 = ct{471};
t6954 = ct{472};
t6960 = ct{473};
t6977 = ct{474};
t6983 = ct{475};
t6984 = ct{476};
t6985 = ct{477};
t6989 = ct{478};
t6990 = ct{479};
t6991 = ct{480};
t6994 = ct{481};
t7 = ct{482};
t7000 = ct{483};
t7003 = ct{484};
t7026 = ct{485};
t7035 = ct{486};
t7036 = ct{487};
t7039 = ct{488};
t7040 = ct{489};
t7084 = ct{490};
t7086 = ct{491};
t7087 = ct{492};
t7095 = ct{493};
t7096 = ct{494};
t7100 = ct{495};
t7103 = ct{496};
t7104 = ct{497};
t712 = ct{498};
t7127 = ct{499};
t7128 = ct{500};
t7129 = ct{501};
t7130 = ct{502};
t7133 = ct{503};
t7134 = ct{504};
t7194 = ct{505};
t72 = ct{506};
t7204 = ct{507};
t7206 = ct{508};
t7207 = ct{509};
t7208 = ct{510};
t724 = ct{511};
t7242 = ct{512};
t7243 = ct{513};
t7245 = ct{514};
t7246 = ct{515};
t7247 = ct{516};
t7254 = ct{517};
t7255 = ct{518};
t7268 = ct{519};
t7270 = ct{520};
t7274 = ct{521};
t7276 = ct{522};
t73 = ct{523};
t7327 = ct{524};
t7331 = ct{525};
t7332 = ct{526};
t7336 = ct{527};
t7340 = ct{528};
t7346 = ct{529};
t7348 = ct{530};
t7349 = ct{531};
t7350 = ct{532};
t7362 = ct{533};
t7363 = ct{534};
t7366 = ct{535};
t7367 = ct{536};
t7368 = ct{537};
t7369 = ct{538};
t7371 = ct{539};
t7372 = ct{540};
t7373 = ct{541};
t7374 = ct{542};
t7375 = ct{543};
t7376 = ct{544};
t7377 = ct{545};
t7378 = ct{546};
t7379 = ct{547};
t7380 = ct{548};
t7381 = ct{549};
t7382 = ct{550};
t7383 = ct{551};
t7384 = ct{552};
t7385 = ct{553};
t7390 = ct{554};
t7391 = ct{555};
t7392 = ct{556};
t7393 = ct{557};
t7394 = ct{558};
t7395 = ct{559};
t7396 = ct{560};
t7398 = ct{561};
t7399 = ct{562};
t7402 = ct{563};
t7403 = ct{564};
t742 = ct{565};
t7423 = ct{566};
t7425 = ct{567};
t7426 = ct{568};
t7427 = ct{569};
t7428 = ct{570};
t7429 = ct{571};
t7430 = ct{572};
t7433 = ct{573};
t7439 = ct{574};
t7440 = ct{575};
t7446 = ct{576};
t7447 = ct{577};
t7448 = ct{578};
t7453 = ct{579};
t7459 = ct{580};
t7463 = ct{581};
t7468 = ct{582};
t7476 = ct{583};
t7477 = ct{584};
t7481 = ct{585};
t7482 = ct{586};
t7485 = ct{587};
t7486 = ct{588};
t7487 = ct{589};
t7488 = ct{590};
t7490 = ct{591};
t7491 = ct{592};
t7492 = ct{593};
t7493 = ct{594};
t7496 = ct{595};
t7498 = ct{596};
t7499 = ct{597};
t7500 = ct{598};
t7501 = ct{599};
t7503 = ct{600};
t7507 = ct{601};
t7509 = ct{602};
t7510 = ct{603};
t7511 = ct{604};
t7512 = ct{605};
t7513 = ct{606};
t7515 = ct{607};
t7516 = ct{608};
t7517 = ct{609};
t7519 = ct{610};
t7521 = ct{611};
t7522 = ct{612};
t7523 = ct{613};
t7524 = ct{614};
t7525 = ct{615};
t7526 = ct{616};
t7527 = ct{617};
t7529 = ct{618};
t7530 = ct{619};
t7531 = ct{620};
t7533 = ct{621};
t7534 = ct{622};
t7536 = ct{623};
t7537 = ct{624};
t7538 = ct{625};
t7541 = ct{626};
t7542 = ct{627};
t7543 = ct{628};
t7546 = ct{629};
t7548 = ct{630};
t7549 = ct{631};
t7550 = ct{632};
t7552 = ct{633};
t7554 = ct{634};
t7555 = ct{635};
t7562 = ct{636};
t7563 = ct{637};
t7565 = ct{638};
t7587 = ct{639};
t7597 = ct{640};
t7599 = ct{641};
t8 = ct{642};
t825 = ct{643};
t827 = ct{644};
t845 = ct{645};
t866 = ct{646};
t869 = ct{647};
t874 = ct{648};
t877 = ct{649};
t881 = ct{650};
t899 = ct{651};
t9 = ct{652};
t90 = ct{653};
t903 = ct{654};
t91 = ct{655};
t919 = ct{656};
t926 = ct{657};
t932 = ct{658};
t947 = ct{659};
t957 = ct{660};
t958 = ct{661};
t968 = ct{662};
t970 = ct{663};
t972 = ct{664};
t984 = ct{665};
t985 = ct{666};
t998 = ct{667};
et903 = t6.*t7.*t8.*t9.*(-8.090164539562037e-7);
et904 = t2.*t4.*t5.*t190.*1.488468502176114e-6;
et905 = t2.*t4.*t9.*t190.*8.090164539562037e-7;
et906 = t4.*t5.*t6.*t190.*6.139979878798348e-6;
et907 = t4.*t6.*t9.*t190.*3.337218585173762e-6;
et908 = t4.*t5.*t34.*t191.*(-1.501384677893902e-29)+t4.*t9.*t34.*t191.*1.968873329708317e-29;
et909 = t5.*t8.*t34.*t191.*(-2.079476307604284e-23)+t8.*t9.*t34.*t191.*3.825923403355188e-23;
et910 = t2.*t5.*t7.*t34.*t191.*1.044940105312709e-22;
et911 = t2.*t7.*t9.*t34.*t191.*(-1.92253250945964e-22);
et912 = t5.*t6.*t7.*t34.*t191.*4.310411145274163e-22;
et913 = t6.*t7.*t9.*t34.*t191.*(-7.930507704503114e-22);
et914 = t7439+t7521+t7522+t7531+t7554+t7555-(t8.*t7331)./2.0-(t2096.*t7130)./2.0-(t2121.*t7129)./2.0+(t3523.*t6821)./2.0+(t3444.*t7130)./2.0+(t3515.*t7129)./2.0+(t4.*t5.*(-t5744+t6232+t6248+t6303+t6322+t6952+t6960+t6983+t6991))./2.0-t5.*t8.*(t5709-t6255+t6282+t6296-t7003+t6216.*(t6218+t5.*(t3136-t5691)).*1.40259855e-11).*(3.0./1.0e+3);
et915 = t4.*t9.*(t6197.*3.383302988283333e-6-t6231+t6954+t6985-t6990+t6216.*(t6218+t5.*(t3136-t5691)).*1.246862701090643e-6).*(-1.0./2.0)+(t4.*t5.*(-t6235+t6248+t6952+t6983-t6989+t6216.*(t6218+t5.*(t3136-t5691)).*1.744166498897461e-6))./2.0-t5.*t8.*t7134.*(3.0./1.0e+3);
et916 = t8.*t9.*t7133.*(-3.0./1.0e+3)+t8.*t9.*t7204.*(3.0./1.0e+3)+(t4.*t9.*t7366)./2.0;
et917 = t257+t278+t358+t372+t374+t428+t434+t436+t445+t448+t458+t460+t477+t486+t508+t510+t512+t522+t535+t547+t561+t587+t592+t596+t612+t827+t899+t958+t972-t7373-t7375-t7378-t7403-t7429-t7430+t7440+t7463-t7515-t7516+t7517+t7519-t7538;
et918 = (t7362.*(t6313+(t91.*t5824.*(t6218+t5.*(t3136-t5691)))./1.316403645856965e+67+(t5824.*t6470.*(t29-t30))./1.316403645856965e+67))./2.0;
et919 = (t8.*(-t5943+t6170-t6177+t6179+t6189-t6605+t6831.*3.146556677756745e-13+t6847-t6849+t6865+t6898+t6921-t6922+t6216.*(t5670+t4.*(t1458-t5665)).*8.40184101230148e-6+t6465.*(t5670+t4.*(t1458-t5665)).*4.126305279697715e-13))./2.0;
et920 = t8.*t9.*(-t5942+t6171+t6183-t6604+t6831.*1.40259855e-11-t6851+t6903+t6924+t6216.*(t5670+t4.*(t1458-t5665)).*1.45270122047331e-4).*(3.0./1.0e+3);
et921 = (t4.*t9.*(-t5944+t6118.*1.246862701090643e-6+t6145+t6146+t6152-t6607+t6831.*3.383302988283333e-6-t6838-t6844-t6856+t6884+t6890+t6909+t6914+t6216.*(t5670+t4.*(t1458-t5665)).*6.293113355513489e-13))./2.0;
et922 = t622+t632+t712+t1503+t1523-t6026+t6035+t6037+t6046-t6711-t6715-t6721-t6743-t6746-t6747+t7206+t7348-t7350+t7367-t7369+t7371-t7485+t7487-t7490-t7512-t7513+t6230.*(t5878+t9.*(t7.*(t3719-t3788)+(t3.*t34.*t191.*(t29-t30))./8.112963841460668e+31)).*2.179051830709965e-7;
et923 = t4.*t9.*(t5709-t6255+t6282+t6296-t7003+t6216.*(t6218+t5.*(t3136-t5691)).*1.40259855e-11).*(3.0./1.0e+3)+t4.*t6465.*(t3136-t5691).*2.179051830709965e-7;
et924 = -t5905+t6048+t6053-t6056+t6060-t6487+t6724+t6727-t6738+t6756+t6758+t6230.*(t5878+t9.*(t7.*(t3719-t3788)+(t3.*t34.*t191.*(t29-t30))./8.112963841460668e+31)).*4.126305279697715e-13-t150.*t5861.*t6468+t4.*t6216.*(t3136-t5691).*8.40184101230148e-6;
et925 = t4.*t6465.*(t3136-t5691).*4.126305279697715e-13;
et926 = t72+t125+t620+t621+t1489+t1508-t5676.*4.35810366141993e-7+t6195.*4.35810366141993e-7+t6196.*8.01825475553694e-7-t6226.*4.35810366141993e-7;
et927 = t6252.*(-4.35810366141993e-7)+t6928.*4.35810366141993e-7+t6935.*4.35810366141993e-7+t6936.*8.01825475553694e-7;
et928 = t6213.*(t6218+t5.*(t3136-t5691)).*(-8.01825475553694e-7)+t73.*t5666+t73.*t6220+t73.*t6239+t9.*t7486+t5.*(t5676.*(-1.246862701090643e-6)+t5730+t5967+t6244+t6249+t6289+t6293+t6307+t6312+t6648+t6656+t6946+t6953+t6977+t6984);
et929 = t258+t277+t287+t356+t361+t372+t422+t433+t444+t448+t453+t475+t485+t493+t514+t524+t533+t561+t586+t592+t603+t610+t827+t899+t958+t972-t7373-t7375-t7378-t7403-t7429-t7430+t7440+t7463-t7515-t7516+t7517+t7519-t7538;
et930 = (t7362.*(t6313+(t91.*t5824.*(t6218+t5.*(t3136-t5691)))./1.316403645856965e+67+(t5824.*t6470.*(t29-t30))./1.316403645856965e+67))./2.0;
et931 = (t8.*(-t5943+t6170-t6177+t6179+t6189-t6605+t6831.*3.146556677756745e-13+t6847-t6849+t6865+t6898+t6921-t6922+t6216.*(t5670+t4.*(t1458-t5665)).*8.40184101230148e-6+t6465.*(t5670+t4.*(t1458-t5665)).*4.126305279697715e-13))./2.0;
et932 = t8.*t9.*(-t5942+t6171+t6183-t6604+t6831.*1.40259855e-11-t6851+t6903+t6924+t6216.*(t5670+t4.*(t1458-t5665)).*1.45270122047331e-4).*(3.0./1.0e+3);
et933 = (t4.*t9.*(-t5944+t6118.*1.246862701090643e-6+t6145+t6146+t6152-t6607+t6831.*3.383302988283333e-6-t6838-t6844-t6856+t6884+t6890+t6909+t6914+t6216.*(t5670+t4.*(t1458-t5665)).*6.293113355513489e-13))./2.0;
et934 = -t6729+t5784.*(t4148+t5.*(t2421-t4158))+(t5824.*t6468.*(t29-t30))./1.316403645856965e+67;
et935 = -(-t5942+t6171+t6183-t6604+t6831.*1.40259855e-11-t6851+t6903+t6924+t6216.*(t5670+t4.*(t1458-t5665)).*1.45270122047331e-4);
et936 = t5961-t6215-t6473+(t91.*t5824.*(t5670+t4.*(t1458-t5665)))./1.316403645856965e+67+(t5824.*t6103.*(t29-t30))./1.316403645856965e+67;
et937 = (t5822.*t6230.*(t29-t30))./1.316403645856965e+67;
et938 = t724+t825+t874+t903+t926+t957+t968+t970+t984+t1004+t1016+t1061+t1081+t1095+t1101+t1108+t1144+t1152+t1155+t1170+t1171+t1174+t1193+t1203+t1207+t1215+t1224+t1245+t1254+t1258+t1285+t1288+t1300+t1301+t1323+t1333+t1344+t1345+t1365+t1377+t1380+t1383+t1388+t1409+t1428+t1440+t1692+t1731+t1769+t1847+t1977+t1981;
et939 = t7402.*(t6313+(t91.*t5824.*(t6218+t5.*(t3136-t5691)))./1.316403645856965e+67+(t5824.*t6470.*(t29-t30))./1.316403645856965e+67);
et940 = -t1429.*(-t5944+t6118.*1.246862701090643e-6+t6145+t6146+t6152-t6607+t6831.*3.383302988283333e-6-t6838-t6844-t6856+t6884+t6890+t6909+t6914+t6216.*(t5670+t4.*(t1458-t5665)).*6.293113355513489e-13)-t1427.*t7534+t7204.*t7276;
et941 = -t7500.*(t6005-t6486+(t5824.*t6230.*(t29-t30))./1.316403645856965e+67)+et934.*et935-t7327.*(et936+et937);
et942 = -t318.*(-t5943+t6170-t6177+t6179+t6189-t6605+t6831.*3.146556677756745e-13+t6847-t6849+t6865+t6898+t6921-t6922+t6216.*(t5670+t4.*(t1458-t5665)).*8.40184101230148e-6+t6465.*(t5670+t4.*(t1458-t5665)).*4.126305279697715e-13);
et943 = t7274.*(t5709-t6255+t6282+t6296-t7003+t6216.*(t6218+t5.*(t3136-t5691)).*1.40259855e-11);
et944 = t7039-t7040-t7095+t7096+t7100-t7103+t7194+t7254+t7255+t7340+t7385+t7395+t7396+t7423+t7425+t7507+t7543+t7546+t7548+(t7000.*(-t6729+t5784.*(t4148+t5.*(t2421-t4158))+(t5824.*t6468.*(t29-t30))./1.316403645856965e+67))./2.0;
et945 = (t7026.*(-t6729+t5784.*(t4148+t5.*(t2421-t4158))+(t5824.*t6468.*(t29-t30))./1.316403645856965e+67))./2.0;
et946 = (t6994.*(t6313+(t91.*t5824.*(t6218+t5.*(t3136-t5691)))./1.316403645856965e+67+(t5824.*t6470.*(t29-t30))./1.316403645856965e+67))./2.0;
et947 = -t3142+t4099+t4103-t4810+t4904+t6118.*2.179051830709965e-7+t6142+t6155+t6158+t6831.*4.00912737776847e-7-t6841-t6842-t6859+t6888+t6891+t6911+t6915+t7374-t7377+t7379+t7426-t7428+t7446-t7468+t7476-t7491-t7492-t7493+t7536;
et948 = (t7346.*(t6313+(t91.*t5824.*(t6218+t5.*(t3136-t5691)))./1.316403645856965e+67+(t5824.*t6470.*(t29-t30))./1.316403645856965e+67))./2.0;
et949 = (t5.*(-t5944+t6118.*1.246862701090643e-6+t6145+t6146+t6152-t6607+t6831.*3.383302988283333e-6-t6838-t6844-t6856+t6884+t6890+t6909+t6914+t6216.*(t5670+t4.*(t1458-t5665)).*6.293113355513489e-13))./2.0;
et950 = (t520.*(t6005-t6486+(t5824.*t6230.*(t29-t30))./1.316403645856965e+67))./2.0;
et951 = t1537+t1540+t1621-t1622+t1642+t1672-t1715+t1719+t1721-t1759-t1770+t1775-t1777+t1870-t1984+t2014+t2034-t2043+t2150+t2165+t2177-t2184-t2203-t2236-t2333-t2341+t2383+t2546-t4153-t4179+t4185-t4190+t4230+t4254+t4255+t4396+t4397+t4412+t4417-t4419-t4420+t4428+t4429-t4440+t4478-t4485-t4506-t4519+t4522-t4530+t4541-t4549+t4557+t4568+t4572+t4596+t4619+t4625+t4648+t4656-t4660-t4727+t4733+t4739+t17.*t1593+t17.*t1704+t18.*t4317;
et952 = t8.*t9.*t199.*(-4.097607815548108e-7)-t5.*t7.*t8.*t199.*2.7046541903611e-13;
et953 = t5.*t8.*t9.*t199.*(-8.376559107229145e-7)-t7.*t9.*t18.*t196.*6.892170885479394e-7;
et954 = t3.*t5.*t34.*t191.*6.288707183017346e-22;
et955 = t4.*t5.*t34.*t191.*(-2.032139097819379e-22);
et956 = t8.*t17.*t19.*t190.*(-1.408936125616489e-6);
et957 = t3.*t9.*t34.*t191.*3.418055254602648e-22;
et958 = t5.*t7.*t34.*t191.*(-2.581060362977273e-29);
et959 = t4.*t9.*t34.*t191.*3.738830062544659e-22;
et960 = t7.*t9.*t34.*t191.*3.384729434006076e-29;
et961 = t5.*t17.*t34.*t191.*(-2.125369829239315e-23);
et962 = t3.*t4.*t5.*t34.*t191.*6.577221276854549e-23;
et963 = t3.*t4.*t9.*t34.*t191.*3.57486922061625e-23;
et964 = t3.*t5.*t8.*t34.*t191.*(-3.384729434006076e-29);
et965 = t3.*t8.*t9.*t34.*t191.*(-2.581060362977273e-29);
et966 = t5.*t7.*t8.*t34.*t191.*3.418055254602648e-22;
et967 = t7.*t8.*t9.*t34.*t191.*(-6.288707183017346e-22);
et968 = t17.*t18.*t24.*t34.*t191.*(-6.080728160647903e-23);
et969 = t4.*t5.*t8.*t17.*t34.*t191.*(-1.534519861952243e-29);
et970 = t5.*t9.*t17.*t18.*t34.*t191.*(-7.993777824483687e-23);
et971 = -dq6.*(dq5.*(et865+et866+et867)+dq2.*(et868+et869+et870)+dq4.*(et914+et915+et916)+dq1.*(et882+et883+et884+et885+et886+et887+et888+et889+et890+et891+et892+et893+et894+et895+et896+et897+et898+et899+et900+et901+et902+et903+et904+et905+et906+et907+et908+et909+et910+et911+et912+et913)-dq3.*(et875+et876+et877+et878+et879+et880+et881)+dq6.*(et871+et872));
et972 = dq2.*(t7550+dq1.*t7549+dq3.*t7599-dq5.*t7597-dq4.*(t5845-t5951+t5954+t5973-t6276+t6546+t6548-t6557-t6562+t7245-t7332+t7383-t7393-t7394-t7398-t7399+t7481+t7523+t7525+(t3444.*(t4148+t5.*(t2421-t4158)))./2.0+(t7511.*(t4148+t5.*(t2421-t4158)))./2.0+(t6352.*(t5709-t6255+t6282+t6296-t7003+t6216.*(t6218+t5.*(t3136-t5691)).*1.40259855e-11))./2.0))+dq1.*(t7550+t7565-dq4.*t7087+dq5.*t7104-dq3.*t7587);
et973 = -dq4.*(dq3.*(et917+et918+et919+et920+et921)+dq4.*(t90+t113+t131+t144+t148+t156+t158+t171+t185-t8.*(et924+et925)+t5.*t8.*t7362.*(3.0./5.0e+2)-t8.*t9.*t7363.*(3.0./5.0e+2)+t4.*t5.*t7511-t4.*t9.*t7510)+dq1.*t7087-dq2.*(t742+t845+t866+t869+t877+t881+t919+t932+t947+t985+t998+t1031+t1075+t1184+t1213+t1227+t1661+t1831+t1858+t2132+t3321+t3407+t3409+t3430+t3450+t3463+t3468+t3475+t3485+t3490+t3496+t3499+t3507+t3513+t3522+t3526+t3531+t3543+t3569+t3583+t3585+t3618+t3658+t3734+t3738+t3843+t3869+t3871+t3992+t4232+t4369+t4436+t4556+t7246+t7247+t7332+t7384+t7393+t7394+t7398+t7399+t7482+t7524+t7526+t7527)+dq6.*(t7439+t7521+t7522+t7531+t7554+t7555)-dq5.*(et922+et923));
et974 = dq5.*(dq1.*t7104-dq4.*(-t115-t132-t2390-t2395+t3606+t3757+t6026+t6042+t6044+t6047+t6711+t6714+t6715+t6721+t6743+t6746+t6747+t6753+t7207+t7208+t7349+t7350+t7368+t7369+t7372+t7485+t7488+t7490+t7512+t7513)-dq2.*(t4148.*(-4.00912737776847e-7)+t5275+t5718+t5738+t7035+t7036+t7084+t7086+t7242+t7243+t7336+t7381+t7382+t7390+t7391+t7392+t7433+t7496+t7498+t7499)-dq3.*(t302+t309+t371+t379+t427+t452+t6147+t6162+t6164+t6165+t6841+t6842+t6859+t6860+t6892+t6894+t6916+t6918+t7127+t7128+t7268+t7270+t7376+t7377+t7380+t7427+t7428+t7447+t7448+t7468+t7477+t7491+t7492+t7493+t7533+t7537)+dq5.*(et926+et927+et928)+dq6.*(t7459+t7501+t7503+t7509+t7541+t7542));
et975 = dq3.*(-dq4.*(et929+et930+et931+et932+et933)+dq3.*(et938+et939+et940+et941+et942+et943)+dq2.*(et944+et945+et946)+dq5.*(et947+et948+et949+et950)-dq1.*(et951+et952+et953+et954+et955+et956+et957+et958+et959+et960+et961+et962+et963+et964+et965+et966+et967+et968+et969+et970)+dq6.*(t7453+t7529+t7530+t7552+t7562+t7563));
C_dq = [et294+et295+et296;et341+et342+et343;et627+et628+et629+et630;et732+et733+et734;et862+et863+et864;et971+et972+et973+et974+et975];
end
